simulink model "inverted_pendulum"  (R2023a)
settings: Solver=VariableStepAuto  StartTime=0.0  StopTime=10.0  RelTol=1e-3
values from neighbouring files (symbols this model uses):
  a = 1/(M+m)    (= 0.1)    [chap5_2plant.m]    (also in chap5_3plant.m)
  g = 9.8    [Robot_plant.m]    (also in adaptive_rbf_nonlinear_system_plant.m; chap5_2plant.m; chap5_3plant.m; control_law_adaptive_rbf_nonlinear_system.m)
  l = 0.5    [adaptive_rbf_nonlinear_system_plant.m]    (also in chap5_2plant.m; chap5_3plant.m; control_law_adaptive_rbf_nonlinear_system.m)
  m = 0.1    [adaptive_rbf_nonlinear_system_plant.m]    (also in adaptive_rbf_with_unknown_parameter_plant.m = 133; chap5_2plant.m = 2; chap5_3plant.m = 2; control_law_adaptive_rbf_nonlinear_system.m)
undefined symbols (not defined in the file or in its folder): magnitude
libraries: simulink_extras x1
settings Model: Creator=ACCENT  LastModifiedBy=ACCENT

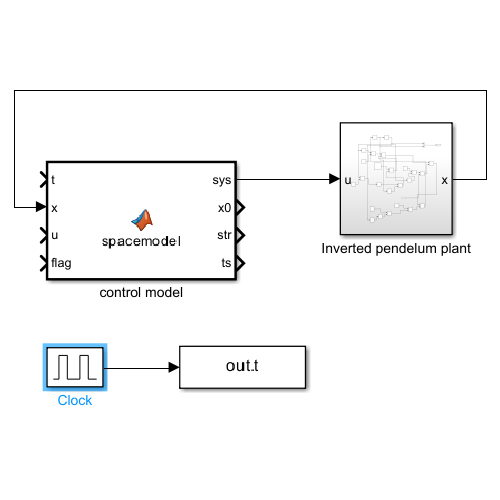
[thumbnail: Simulink's stored preview of the top-level diagram]
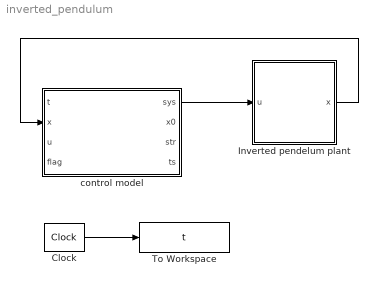
== system inverted_pendulum ==
  Clock : simulink_extras/Flip Flops/Clock  period=5
  Inverted pendelum plant : Subsystem
  To Workspace : ToWorkspace  VariableName=t  SaveFormat=Timeseries  SampleTime=-1
  control model : MATLAB Function  TreatAsAtomicUnit=on
  wires:
  Inverted pendelum plant/1(x) -> control model/2(x)
  control model/1(sys) -> Inverted pendelum plant/1(u)
  Clock/1 -> To Workspace/1

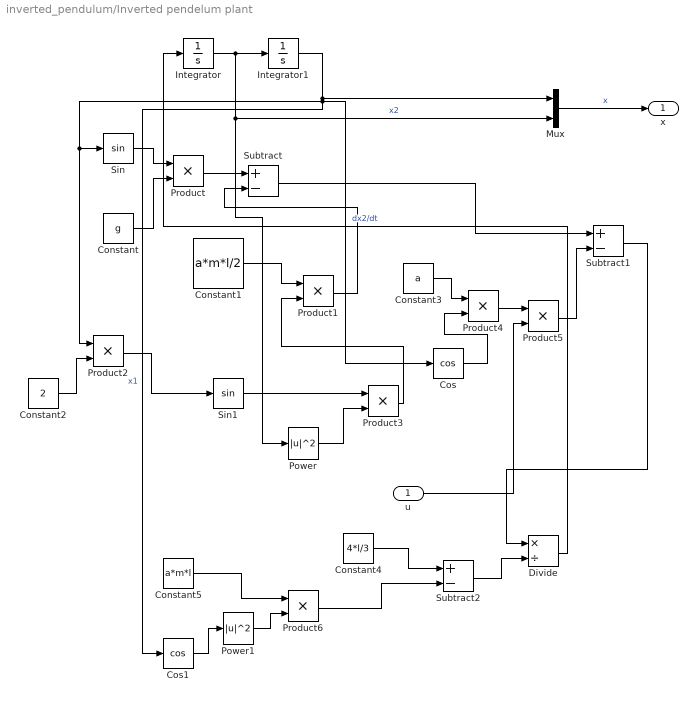
== system inverted_pendulum/Inverted pendelum plant ==
  u : Inport
  Constant : Constant  Value=g
  Constant1 : Constant  Value=a*m*l/2
  Constant2 : Constant  Value=2
  Constant3 : Constant  Value=a
  Constant4 : Constant  Value=4*l/3
  Constant5 : Constant  Value=a*m*l
  Cos : Trigonometry  Operator=cos
  Cos1 : Trigonometry  Operator=cos
  Divide : Product  Inputs=*/
  Integrator : Integrator
  Integrator1 : Integrator
  Mux : Mux  Inputs=2
  Power : Math  Operator=magnitude^2
  Power1 : Math  Operator=magnitude^2
  Product{,1..6} (7 alike) : Product
  Sin : Trigonometry
  Sin1 : Trigonometry
  Subtract : Sum  Inputs=+-
  Subtract1 : Sum  Inputs=+-
  Subtract2 : Sum  Inputs=+-
  x : Outport
  wires:
  Cos/1 -> Product4/2
  Integrator1/1 -> Mux/1, Cos1/1, Product2/1, Sin/1, Cos/1  "x1"
  Product/1 -> Subtract/1
  Divide/1 -> Integrator/1  "dx2/dt"
  Constant1/1 -> Product1/1
  Constant4/1 -> Subtract2/1
  Integrator/1 -> Mux/2, Power/1, Integrator1/1  "x2"
  Power/1 -> Product3/2
  Sin/1 -> Product/1
  Product1/1 -> Subtract/2
  Subtract/1 -> Subtract1/1
  Constant5/1 -> Product6/1
  Product3/1 -> Product1/2
  Constant/1 -> Product/2
  Product2/1 -> Sin1/1
  u/1 -> Product5/2
  Constant3/1 -> Product4/1
  Product5/1 -> Subtract1/2
  Sin1/1 -> Product3/1
  Constant2/1 -> Product2/2
  Product4/1 -> Product5/1
  Subtract1/1 -> Divide/1
  Subtract2/1 -> Divide/2
  Cos1/1 -> Power1/1
  Product6/1 -> Subtract2/2
  Power1/1 -> Product6/2
  Mux/1 -> x/1  "x"

== matlab function inverted_pendulum/control model ==
  data: sys output; x0 output; str output; ts output; t input; x input; u input; flag input

function [sys,x0,str,ts] = spacemodel(t,x,u,flag)
switch flag,
case 0,
[sys,x0,str,ts]=mdlInitializeSizes;
case 3,
sys=mdlOutputs(t,x,u);
case {2,4,9}
sys=[];
otherwise
error(['Unhandled flag = ',num2str(flag)]);
end
function [sys,x0,str,ts]=mdlInitializeSizes
sizes = simsizes;
sizes.NumContStates = 0;
sizes.NumDiscStates = 0;
sizes.NumOutputs = 1;
sizes.NumInputs = 2;
sizes.DirFeedthrough = 1;
sizes.NumSampleTimes = 1;
sys = simsizes(sizes);
x0 = [];
str = [];
ts = [0 0];
function sys=mdlOutputs(t,x,u)
x=[u(1);u(2)];
loadK_file;
ut1=K1*x;
ut2=K2*x;
ut3=K3*x;
ut4=K4*x;
L1=-pi;L2=pi;
L=L2-L1;
h=pi/2;
N=L/h;
fori=1:N+1
e(i)=L1+L/N*(i-1);
end
% h1
h1=trimf(x(1),[e(2),e(3),e(4)]); %Rule 1:x1 is to zero
% h2, Rule 2: x1 is about +-pi/2,but smaller
if x(1)<=0
h2=trimf(x(1),[e(2),e(2),e(3)]);
else
h2=trimf(x(1),[e(3),e(4),e(4)]);
end
% h3, Rule 3: x1 is about +-pi/2,but bigger
if x(1)<0
h3=trimf(x(1),[e(1),e(2),e(2)]);
else
h3=trimf(x(1),[e(4),e(4),e(5)]);
end
% h4, Rule 4: x1 is about +-pi
if x(1)<0
h4=trimf(x(1),[e(1),e(1),e(2)]);
else
h4=trimf(x(1),[e(4),e(5),e(5)]);
end
h1+h2+h3+h4;
ut=(h1*ut1+h2*ut2+h3*ut3+h4*ut4)/(h1+h2+h3+h4);
sys(1)=ut;
end
end
